simulink model "Super5_tmp"  (Simulink 8.3)
settings: Solver=ode45  StartTime=0.0  StopTime=10.0  RelTol=1e-3
settings Model: Creator=scaife  LastModifiedBy=bourbouh  CovSFcnEnable=on  ExtModeAutoUpdateStatusClock=off
settings DataIOCC: SignalLoggingName=sigsOut
settings DebuggingCC: SaveWithParameterizedLinksMsg=none  SignalResolutionControl=TryResolveAllWithWarning  SolverPrmCheckMsg=none  MultiTaskDSMMsg=warning  MultiTaskCondExecSysMsg=none  FrameProcessingCompatibilityMsg=error  StateNameClashWarn=none
settings HardwareCC: TargetUnknown=on
settings SFSimCC: SimParseCustomCode=off
settings GRTTargetCC: GeneratePreprocessorConditionals=Use local settings

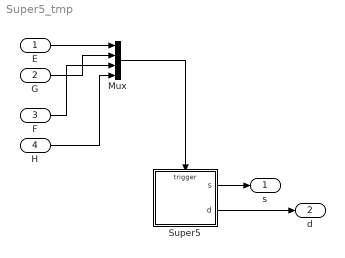
== system Super5_tmp ==
  E : Inport
  G : Inport  Port=2
  F : Inport  Port=3
  H : Inport  Port=4
  Mux : Mux
  Super5 : Stateflow chart  TreatAsAtomicUnit=on
      settings: PermitHierarchicalResolution=ParametersOnly
  s : Outport
  d : Outport  Port=2
  wires:
  E/1 -> Mux/1
  G/1 -> Mux/2
  F/1 -> Mux/3
  H/1 -> Mux/4
  Mux/1 -> Super5/Trigger
  Super5/1(s) -> s/1
  Super5/2(d) -> d/1

== stateflow chart Super5 ==
  state A
    en: s = 1;
    du: d++;
    state A1
      en: s = 2;
      du: d++;
    (default) -> A1
  state B
    en: s = 3;
    du: d++;
    state B1
      en: s = 4;
      du: d++;
    (default) -> B1
  state D
    en: s = 5;
    du: d++;
    state D1
      en: s = 6;
      du: d++;
    (default) -> D1
  state C
    en: s = 7;
    du: d++;
    state C1
      en: s = 8;
      du: d++;
    (default) -> C1
  (default) -> A
  A -> B [order 1] : G
  A1 -> B1 [order 1] : E
  B1 -> A1 [order 2] : F
  D1 -> A1 [order 1] : E
  A1 -> D1 [order 2] : F
  C1 -> B1 [order 1] : F
  B1 -> C1 [order 1] : E
  B -> A [order 2] : H
  A -> D [order 2] : H
  D -> A [order 1] : G
  C -> B [order 1] : H
  B -> C [order 1] : G
  D -> C [order 2] : H
  D1 -> C1 [order 2] : F
  C1 -> D1 [order 2] : E
  C -> D [order 2] : G
  data: s output double; d output double
  events: E input EITHER_EDGE_EVENT; G input EITHER_EDGE_EVENT; F input EITHER_EDGE_EVENT; H input EITHER_EDGE_EVENT
